simulink model "Adaptive_Cruise_Control"  (R2018a)
settings: Solver=VariableStepAuto  StartTime=0.0  StopTime=10.0  RelTol=1e-3
values from neighbouring files (symbols this model uses):
  F_aero = 1/(2*m_Follower) * Ro_A_Cd    (= 0.000326666666667)    [ACC_DATA.m]
  F_grav = g * sin(theta)    [ACC_DATA.m]
  F_res = Cr * g * cos(theta)    [ACC_DATA.m]
  Kb = 0.005    [ACC_DATA.m]
  Kc = 1    [ACC_DATA.m]
  r = 0.326    [ACC_DATA.m]
  Rf = 3.28    [ACC_DATA.m]
  Tmax = 528.7 + 0.152*Ne - 0.0000217*Ne^2    (= 789.5)    [ACC_DATA.m]
undefined symbols (not defined in the file or in its folder): Ct, m, Rt
settings Model: Creator=Talha Rao  LastModifiedBy=Talha Rao

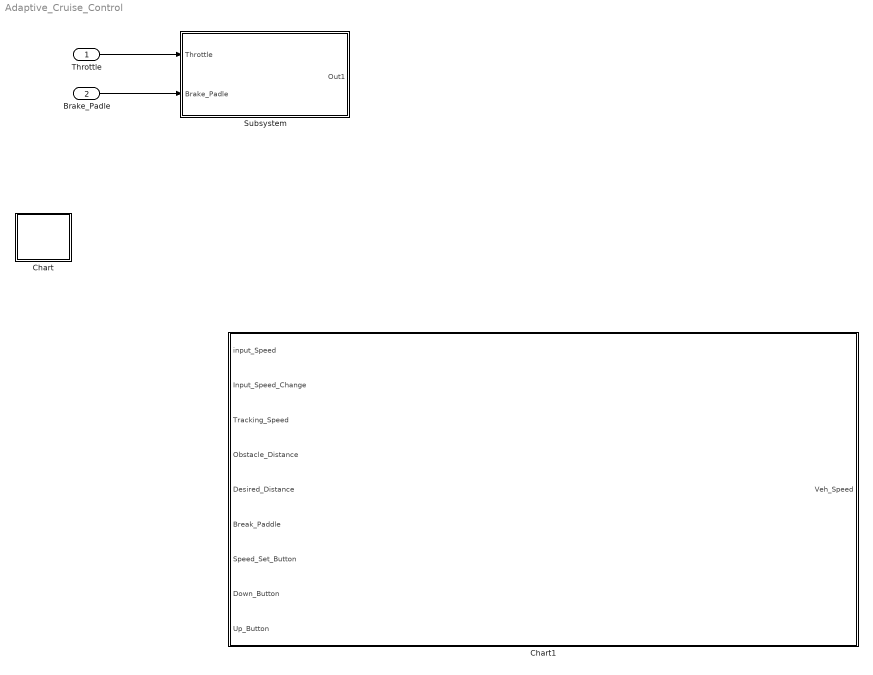
== system Adaptive_Cruise_Control ==
  Throttle : Inport
  Brake_Padle : Inport  Port=2
  Chart : Stateflow chart  TreatAsAtomicUnit=on
  Chart1 : Stateflow chart  TreatAsAtomicUnit=on
  Subsystem : Subsystem
  wires:
  Throttle/1 -> Subsystem/1(Throttle)
  Brake_Padle/1 -> Subsystem/2(Brake_Padle)

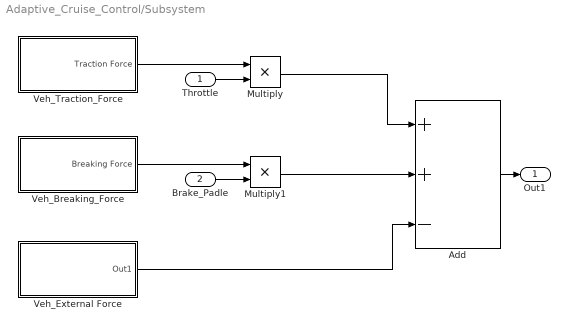
== system Adaptive_Cruise_Control/Subsystem ==
  Throttle : Inport
  Brake_Padle : Inport  Port=2
  Add : Sum  Inputs=++-
  Multiply : Product
  Multiply1 : Product
  Veh_Breaking_Force : Subsystem
  Veh_External Force : Subsystem
  Veh_Traction_Force : Subsystem
  Out1 : Outport
  wires:
  Veh_External Force/1(Out1) -> Add/3
  Brake_Padle/1 -> Multiply1/2
  Veh_Breaking_Force/1("Breaking Force ") -> Multiply1/1
  Throttle/1 -> Multiply/2
  Add/1 -> Out1/1
  Multiply1/1 -> Add/2
  Multiply/1 -> Add/1
  Veh_Traction_Force/1(Traction Force) -> Multiply/1

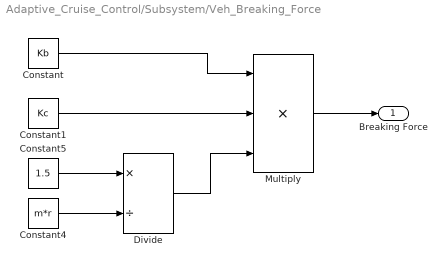
== system Adaptive_Cruise_Control/Subsystem/Veh_Breaking_Force ==
  Constant : Constant  Value=Kb
  Constant1 : Constant  Value=Kc
  Constant4 : Constant  Value=m*r
  Constant5 : Constant  Value=1.5
  Divide : Product  Inputs=*/
  Multiply : Product  Inputs=3
  "Breaking Force " : Outport
  wires:
  Multiply/1 -> "Breaking Force "/1
  Constant4/1 -> Divide/2
  Constant1/1 -> Multiply/2
  Constant/1 -> Multiply/1
  Constant5/1 -> Divide/1
  Divide/1 -> Multiply/3

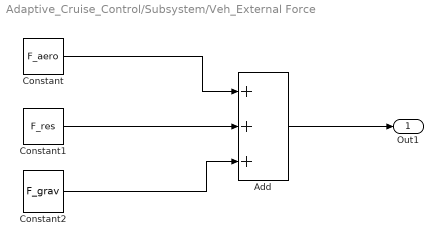
== system Adaptive_Cruise_Control/Subsystem/Veh_External Force ==
  Add : Sum  Inputs=+++
  Constant : Constant  Value=F_aero
  Constant1 : Constant  Value=F_res
  Constant2 : Constant  Value=F_grav
  Out1 : Outport
  wires:
  Add/1 -> Out1/1
  Constant/1 -> Add/1
  Constant1/1 -> Add/2
  Constant2/1 -> Add/3

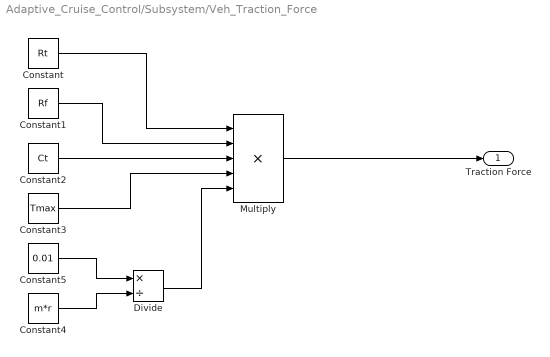
== system Adaptive_Cruise_Control/Subsystem/Veh_Traction_Force ==
  Constant : Constant  Value=Rt
  Constant1 : Constant  Value=Rf
  Constant2 : Constant  Value=Ct
  Constant3 : Constant  Value=Tmax
  Constant4 : Constant  Value=m*r
  Constant5 : Constant  Value=0.01
  Divide : Product  Inputs=*/
  Multiply : Product  Inputs=5
  Traction Force : Outport
  wires:
  Constant/1 -> Multiply/1
  Constant4/1 -> Divide/2
  Constant1/1 -> Multiply/2
  Constant5/1 -> Divide/1
  Constant3/1 -> Multiply/4
  Divide/1 -> Multiply/5
  Constant2/1 -> Multiply/3
  Multiply/1 -> Traction Force/1

== stateflow chart Adaptive_Cruise_Control/Chart1 ==
  state CRUISE_CONTROL_OFF
    Veh_Speed = input_Speed;
  state NORMAL_CRUISE_CONTROL_ON
    state UP_BUTTON_PRESSED
      Veh_Speed = Veh_Speed + 5;
    state DOWN_BUTTON_PRESSED
      Veh_Speed = Veh_Speed - 5;
    state Cruise_Control_ON
      Veh_Speed = Veh_Speed;
    state REFRESH_TO_REFRENCE
      Veh_Speed = input_Speed;
    (default) -> Cruise_Control_ON : {Veh_Speed = input_Speed}
    Cruise_Control_ON -> DOWN_BUTTON_PRESSED [order 2] : [Down_Button>0]
    Cruise_Control_ON -> UP_BUTTON_PRESSED [order 1] : [Up_Button > 0]
    DOWN_BUTTON_PRESSED -> Cruise_Control_ON
    UP_BUTTON_PRESSED -> Cruise_Control_ON
    REFRESH_TO_REFRENCE -> Cruise_Control_ON
    Cruise_Control_ON -> REFRESH_TO_REFRENCE [order 3] : [Input_Speed_Change > 0]
  state ACTUATOR_LOGIC
  state CRUISE_CONTROL_TRACKING_MODE_ON
    Veh_Speed = Tracking_Speed;
  (default) -> CRUISE_CONTROL_OFF [order 1]
  CRUISE_CONTROL_TRACKING_MODE_ON -> CRUISE_CONTROL_OFF [order 2] : [Break_Paddle > 0 ]
  CRUISE_CONTROL_OFF -> NORMAL_CRUISE_CONTROL_ON : [Break_Paddle == 0 && Veh_Speed > 30 && Speed_Set_Button > 0]
  (default) -> CRUISE_CONTROL_OFF [order 2] : [Break_Paddle == 1 || Veh_Speed < 30 ]
  CRUISE_CONTROL_TRACKING_MODE_ON -> NORMAL_CRUISE_CONTROL_ON [order 1] : [Obstacle_Distance > Desired_Distance ]
  NORMAL_CRUISE_CONTROL_ON -> CRUISE_CONTROL_TRACKING_MODE_ON : [Obstacle_Distance < Desired_Distance ]
  data: input_Speed input; Input_Speed_Change input; Tracking_Speed input; Obstacle_Distance input; Desired_Distance input; Break_Paddle input; Speed_Set_Button input; Down_Button input; Up_Button input; Veh_Speed output

== stateflow chart Adaptive_Cruise_Control/Chart ==
  state UP_BUTTON_PRESSED
    Veh_Speed = Veh_Speed + 5;
  state DOWN_BUTTON_PRESSED
    Veh_Speed = Veh_Speed - 5;
  state Cruise_Control_ON
    Veh_Speed = Veh_speed;
  (default) -> Cruise_Control_ON
  Cruise_Control_ON -> DOWN_BUTTON_PRESSED [order 2] : [Down_Button>0]
  Cruise_Control_ON -> UP_BUTTON_PRESSED [order 1] : [Up_Button > 0]
  DOWN_BUTTON_PRESSED -> Cruise_Control_ON
  UP_BUTTON_PRESSED -> Cruise_Control_ON
